simulink model "VehicleDynamics_PathPlanning"  (R2023a)
settings: Solver=FixedStepAuto  StartTime=0.0  StopTime=150  FixedStep=1e-3  RelTol=1e-3
PreLoadFcn:
  | addpath(genpath(pwd));
  | 
  | % ======================================================================= %
  | %% Physics Paramters
  | 
  | g = 9.81;           % [m/s2]
  | rho_air = 1.2;      % [kg/m3]
  | 
  | % ======================================================================= %
  | %% Tire Paramters
  | 
  | mu = 1;           % [-]
  | 
  | B_f = 3.12;
  | B_r = 2.91;
  | C_f = 2.23;
  | C_r = 2.23;
  | D_f = 0.72;
  | D_r = 1.21;
  | E_f = 0.23;
  | E_r = 0.92;
  | 
  | % ======================================================================= %
  | %% Motor Paramters
  | 
  | P_max = 7.6*100;        % [W]
  | 
  | w_l = 1000;           % [RPM]
  | 
  | Motor_Param.eDrivetrain       = 0.8*0.8*0.3;    % [-] %  \eta_i*\eta_d*correction_term
  | 
  | GR1 = 3.3250;         % 84/48*38/20
  | GR2 = 2.90;
  | 
  | % ======================================================================= %
  | %% Car Paramters
  | 
  | widthCar           = 0.31;           % [m]
  | heightCar          = 0.115;          % [m]
  | C_Drag             = 0.7;            % [m]
  | 
  | Car_Param.lTrackWidth         = 0.165;          % [m]
  | l_wb          = 0.3070;           % [m]
  | 
  | mWheel               = 0.03;           % [kg]
  | rWheel               = 0.03;           % [m]
  | I_wheel              = 2.0760e-05;     % [kgm2] % 1/2*mWheel*(rWheel^2+0.022^2)
  | reffWheel            = 0.1885;         % [m]    % rWheel*2*pi
  | 
  | mCar                = 3.31;            % [kg]   % car mass
  | I_z                 = 0.09;            % [kgm2] % 1/12*mCar*(lTrackWidth^2+lWheelbase^2)
  | 
  | h_cg     = 0.02;           % [m]
  | 
  | % ======================================================================= %
  | %% Track Select
  | 
  | NTrack = 1;  % Austin Min Curv
  | % NTrack = 2;  % Austin Shortest Path
  | 
  | % NTrack = 3;  % Silverstone Min Curv
  | % NTrack = 4;  % Silverstone Shortest Path
  | 
  | run TrackData.m
  | Track_Param.rTrajOpt = 0.005; %0.005;
  | 
  | % ======================================================================= %
  | %% Offline Trajectory Optimization
  | 
  | % run Trajectory_Optimizer.m
  | % Track_Param.xTrack=xTraj;
  | % Track_Param.yTrack=yTraj;
StopFcn:
  | Data1=out.CarPosition.Data;
  | 
  | figure(2)
  | cmap = colormap(jet);
  | s=scatter(Data1(:,1),Data1(:,2),0.1,Data1(:,4),'.');
  | c=colorbar;
  | ylabel(c,'v_{Car} (m/s)')
  | 
  | hold on
  | plot(xCentre, yCentre, 'k')
  | plot(xRightside,yRigthside,'k--')
  | k=plot(xLeftside ,yLeftside ,'k--');
  | sf=plot(xStartLine,yStartLine,'k-.');
  | 
  | s.Annotation.LegendInformation.IconDisplayStyle = 'off';
  | k.Annotation.LegendInformation.IconDisplayStyle = 'off';
  | sf.Annotation.LegendInformation.IconDisplayStyle = 'off';
  | legend('Track centerline','Track limits')
  | axis off
  | text(0.5,-5,'S/F\rightarrow','HorizontalAlignment','center')
  | % title('Car position and velocity')
  | 
  | clear Data1 cmap s c k sf
values from neighbouring files (symbols this model uses):
  A_frontal = 0.03565    [PathPlanningFinal.mat]
  C_drag = 0.7    [PathPlanningFinal.mat]
  C_RR = 0.01    [PathPlanningFinal.mat]
  eDriveTrain = 0.192    [PathPlanningFinal.mat]
  l_f = 0.162    [PathPlanningFinal.mat]
  l_r = 0.145    [PathPlanningFinal.mat]
  xStartLine = [-0.53 -0.53]    [PathPlanningFinal.mat]    (also in TrackData.m = [X(1),X(1)])
  xTraj = [-3.58492023158 -0.667650571356 2.24958592115 5.16684606266 8.08415362212 11.0015140612 13.9188994094 16.8363143954 19.7537503159 22.6711684367 25.5885689606 28.505984703 ... (1500 elements, 1500x1)]    [PathPlanningFinal.mat]
  yStartLine = [-3.75 3.75]    [PathPlanningFinal.mat]    (also in TrackData.m = Y(1)+1.5*[-lHalfTrackWidth,lHalfTrackWidth])
  yTraj = [-1.92786957575 -4.15585802925 -6.3838214679 -8.6118036214 -10.8398229653 -13.0678839828 -15.2959656084 -17.5240717548 -19.7521960674 -21.9803092429 -24.2084117195 -26.4365288431 ... (1500 elements, 1500x1)]    [PathPlanningFinal.mat]
libraries: simulink x5, dspfdesign x2, drivingvehiclecontroller x1
settings Model: Creator=Rakshit Jangid  LastModifiedBy=Rakshit Jangid
settings DataIOCC: SaveState=on
settings ModelReferenceCC: UpdateModelReferenceTargets=IfOutOfDate  EnableRefExpFcnMdlSchedulingChecks=on
settings RTWCC: BuildConfiguration=Faster Runs

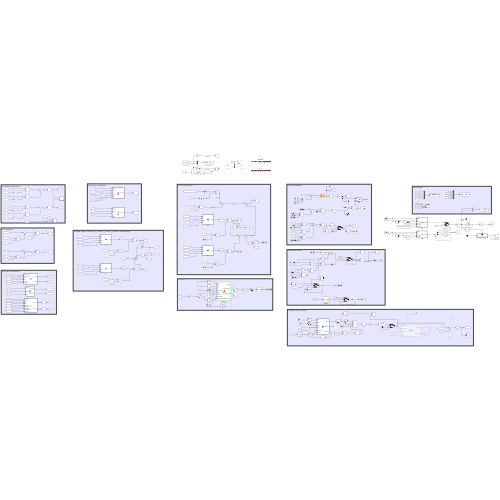
[thumbnail: Simulink's stored preview of the top-level diagram]
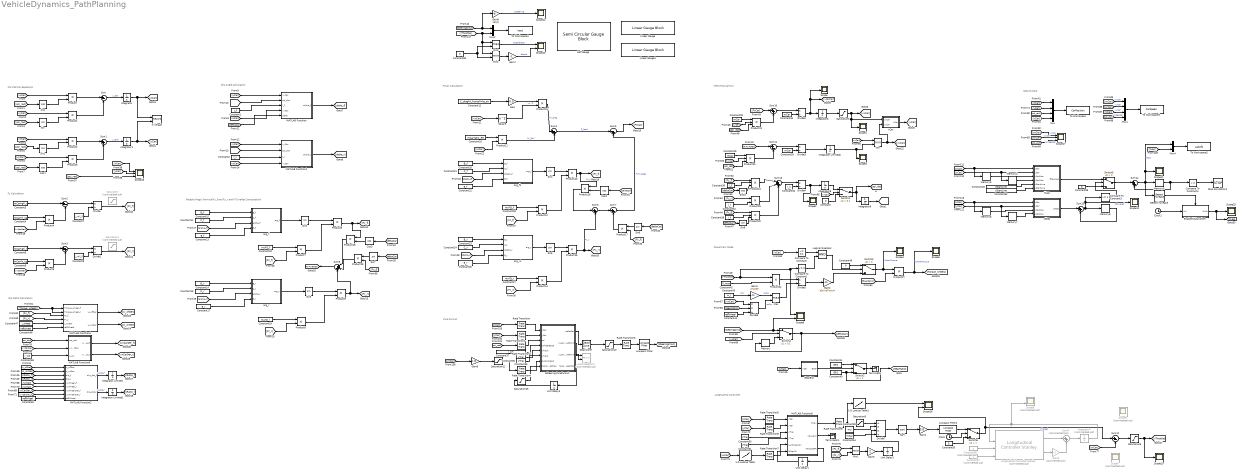
== system VehicleDynamics_PathPlanning ==
  note: Data Output
  note: Pure Pursuit
  note: Longitudinal Controller
  note: Powertrain Model
  note: Vehicle Dynamics
  note: FxCar Calculation
  note: Slip Ratio Calculation
  note: Pacejka Magic Formula(Fy_f and Fy_r and FyTyreNet Computation)
  note: Fz Calculation
  note: Slip Angle Calculation
  note: Car Position Equations
  1-D Lookup Table : Lookup_n-D  NumberOfTableDimensions=1  BreakpointsForDimension1=[7.5, 10, 15, 20]  Table=[5, 10, 25, 40]  ExtrapMethod=Clip  InternalRulePriority=Speed  RndMeth=Simplest
  1-D Lookup Table1 : Lookup_n-D  NumberOfTableDimensions=1  BreakpointsForDimension1=[0,0.04,0.1,0.2,0.3,0.5]*1  Table=[20, 10, 9, 6, 5, 4]  ExtrapMethod=Clip  InternalRulePriority=Speed  RndMeth=Simplest
  Clock : Clock
  Clock1 : Clock
  Compare To Constant : simulink/Logic and Bit Operations/Compare To Constant  relop=<=  const=0.1  OutDataTypeStr=boolean
  Compare To Constant1 : simulink/Logic and Bit Operations/Compare To Constant  relop=<=  const=0  OutDataTypeStr=boolean
  Compare To Constant3 : simulink/Logic and Bit Operations/Compare To Constant  relop=>=  const=1  OutDataTypeStr=boolean
  Compare To Constant4 : simulink/Logic and Bit Operations/Compare To Constant  relop=>  const=2  OutDataTypeStr=boolean
  Constant{,46,59..60} (4 alike) : Constant  Value=0
  Constant1 : Constant  Value=l_f
  Constant10 : Constant  Value=B_f
  Constant11 : Constant  Value=C_f
  Constant12 : Constant  Value=C_drag*A_frontal*rho_air
  Constant13 : Constant  Value=E_f
  Constant14 : Constant  Value=B_r
  Constant15 : Constant  Value=C_r
  Constant16 : Constant  Value=mCar*g*C_RR
  Constant17 : Constant  Value=E_r
  Constant18 : Constant  Value=mu*D_f
  Constant19 : Constant  Value=mu*D_r
  Constant2 : Constant  Value=l_r
  Constant20 : Constant  Value=B_f
  Constant21 : Constant  Value=C_f
  Constant22 : Constant  Value=E_f
  Constant23 : Constant  Value=B_r
  Constant24 : Constant  Value=C_r
  Constant25 : Constant  Value=E_r
  Constant26 : Constant  Value=mu*D_f
  Constant27 : Constant  Value=mu*D_r
  Constant{28..29,33..34,54} (5 alike) : Constant  Value=mCar
  Constant3 : Constant  Value=mCar*g*l_r
  Constant30 : Constant  Value=l_f
  Constant31 : Constant  Value=l_r
  Constant32 : Constant  Value=I_z
  Constant35 : Constant  Value=xTraj
  Constant36 : Constant  Value=yTraj
  Constant37 : Constant  Value=l_wb
  Constant38 : Constant  Value=l_f
  Constant4 : Constant  Value=mCar*h_cg
  Constant40 : Constant  Value=GR1
  Constant41 : Constant  Value=GR2
  Constant42 : Constant  Value=P_max
  Constant43 : Constant  Value=w_l
  Constant44 : Constant  Value=reffWheel
  Constant47 : Constant  Value=I_wheel
  Constant48 : Constant  Value=reffWheel
  Constant49 : Constant  Value=xStartLine
  Constant5 : Constant  Value=reffWheel
  Constant50 : Constant  Value=xTraj
  Constant51 : Constant  Value=yTraj
  Constant52 : Constant  Value=yStartLine
  Constant53 : Constant  Value=mu
  Constant55 : Constant  Value=5
  Constant56 : Constant  Commented=on
  Constant57 : Constant  Commented=on  Value=0
  Constant58 : Constant  Value=l_wb
  Constant6 : Constant  Value=mCar*g*l_f
  Constant7 : Constant  Value=l_r+l_f
  Constant8 : Constant  Value=mCar*h_cg
  Constant9 : Constant  Value=l_r+l_f
  Cos{,1..3} (4 alike) : Trigonometry  Operator=cos
  Dead Zone : DeadZone  LowerValue=-0.5*pi/180  UpperValue=0.5*pi/180
  Detect Increase : simulink/Logic and Bit Operations/Detect Increase  vinit=0.0  OutDataTypeStr=boolean
  Divide{,1..5} (6 alike) : Product  Inputs=*/
  Divide6 : Product  Inputs=**/
  Divide7 : Product  Inputs=/**/
  Enabled Subsystem : Subsystem  TreatAsAtomicUnit=on
  Gain : Gain  Gain=0.5
  Gain1 : Gain  Gain=2*pi/60
  Gain2 : Gain  Gain=eDriveTrain/4
  Gain3 : Gain  Gain=2
  Gain4 : Gain  Gain=0.8
  Gain5 : Gain  Commented=on  Gain=-1
  Gain6 : Gain  Gain=0.25
  Gain7 : Gain  Gain=-1
  Gain8 : Gain  Gain=180/pi
  GearBox : Stateflow chart  TreatAsAtomicUnit=on
  Half Gauge : SemiCircularGaugeBlock  LabelPosition=Bottom  ScaleMin=-5  ScaleMax=5
  Integrator{,1,6,8..9} (5 alike) : Integrator
  Integrator Limited : Integrator  LimitOutput=on  UpperSaturationLimit=10*pi/180  LowerSaturationLimit=-10*pi/180
  Integrator Limited1 : Integrator  LimitOutput=on  UpperSaturationLimit=10*pi/180  LowerSaturationLimit=-10*pi/180
  Integrator Limited2 : Integrator  LimitOutput=on  UpperSaturationLimit=1  LowerSaturationLimit=-1
  Integrator4 : Integrator  Commented=on
  Linear Gauge : LinearGaugeBlock  ScaleMax=1
  Linear Gauge1 : LinearGaugeBlock  ScaleMax=1
  Logical Operator : Logic  AllPortsSameDT=off  OutDataTypeStr=boolean
  Longitudinal Controller Stanley : drivingvehiclecontroller/Longitudinal Controller Stanley  Commented=on  Kp=2.5  Ki=1  SampleTime=0.05  MaxAcceleration=3  MaxDeceleration=6
  LookAheadPoint : Record  Commented=on  FileSettingsInternal="{\"entries\":[{\"content\":{\"excelSettings\":{\"content\":{},\"type\":\"Streamout.ExcelSettings\"}},\"type\":\"Streamout.FileSettingStorage\",\"uuid\":\"\"}],\"packageUris\":[\"http:\\/\\/schema.mathworks.com\\/mf0\\/streamout_blocks\\/R2020a\"],\"version\":\"1.0\"}"  Layout=[1 1]  SignalsInternal="{\"entries\":[{\"content\":{\"signals\":[{\"content\":{\"blockPath\":[],\"dimensions\":[1],\"domain\":\"\",\"lineColor\":\"#a2142f\",\"plots\":[1],\"port\":1,\"signalID\":34,\"signalName\":\"XY Graph:1\"},\"type\":\"RecordBlkView.Signal\",\"uuid\":\"\"},{\"content\":{\"blockPath\":[],\"dimensions\":[1],\"domain\":\"\",\"lineColor\":\"#139fff\",\"plots\":[1],\"port\":2,\"signalID\":37,\"signalName\":\"XY Graph:2\"},\"type\":\"RecordBlkView.Signal\",\"uuid\":\"\"}]},\"type\":\"RecordBlkView.InputSignals\",\"uuid\":\"\"}],\"packageUris\":[\"http:\\/\\/schema.mathworks.com\\/mf0\\/streamout_blocks\\/R2020a\"],\"version\":\"1.0\"}"  VisualizationBindings="{\"xyplotplugin\":{\"info\":[{\"series\":[{\"bindingParametersList\":[{\"parameter\":\"X-Axis\",\"signalID\":34,\"signalName\":\"XY Graph:1\"},{\"parameter\":\"Y-Axis\",\"signalID\":37,\"signalName\":\"XY Graph:2\"}],\"seriesID\":34788}],\"subplotID\":1}]}}"  CompatibilityTag=XY  st=-1
  Lowpass Filter : dspfdesign/Lowpass Filter  FilterType=FIR  DesignForMinimumOrder=on  FilterOrder=50  PassbandFrequency=50  StopbandFrequency=100  PassbandRipple=0.1  StopbandAttenuation=50  SampleRateMode=Specify on dialog  SampleRate=1000  SimulateUsing=Interpreted execution  roundingMode=Floor  coeffsDataTypeStr=fixdt(1,16)
  Lowpass Filter2 : dspfdesign/Lowpass Filter  FilterType=FIR  DesignForMinimumOrder=on  FilterOrder=50  PassbandFrequency=2  StopbandFrequency=10  PassbandRipple=0.1  StopbandAttenuation=50  SampleRateMode=Specify on dialog  SampleRate=1000  SimulateUsing=Interpreted execution  roundingMode=Floor  coeffsDataTypeStr=fixdt(1,16)
  MATLAB Function : MATLAB Function  TreatAsAtomicUnit=on
  MATLAB Function1 : MATLAB Function  TreatAsAtomicUnit=on
  MATLAB Function2 : MATLAB Function  TreatAsAtomicUnit=on
  MATLAB Function4 : MATLAB Function  TreatAsAtomicUnit=on
  MATLAB Function5 : MATLAB Function  TreatAsAtomicUnit=on
  MATLAB Function6 : MATLAB Function  TreatAsAtomicUnit=on
  Max : MinMax  Function=max  Inputs=2
  Memory{,3..4,6..8} (6 alike) : Memory
  Memory5 : Memory  InitialCondition=1
  Min : MinMax  Inputs=2
  Min1 : MinMax  Inputs=2
  Min2 : MinMax  Inputs=2
  Min3 : MinMax  Function=max  Inputs=2
  Mux : Mux
  Mux1 : Mux
  Mux2 : Mux  Inputs=2
  Mux4 : Mux  Inputs=2
  NLap : MATLAB Function  TreatAsAtomicUnit=on
  Product{,1..19,22,25,27} (23 alike) : Product
  Product{20..21,23..24} (4 alike) : Product  Inputs=3
  Rate Transition{,1..2,4..7} (7 alike) : RateTransition  OutPortSampleTime=0.01
  Rate Transition3 : RateTransition  OutPortSampleTime=0.001
  Rate Transition8 : RateTransition  OutPortSampleTime=0.001
  Saturation : Saturate  Commented=on  UpperLimit=mCar*g  LowerLimit=-mCar*g/2
  Saturation1 : Saturate  Commented=on  UpperLimit=mCar*g  LowerLimit=-mCar*g/2
  Saturation10 : Saturate  UpperLimit=26*pi/180  LowerLimit=-26*pi/180
  Saturation12 : Saturate  UpperLimit=5  LowerLimit=1
  Saturation15 : Saturate  UpperLimit=100  LowerLimit=1
  Saturation3 : Saturate  UpperLimit=inf  LowerLimit=0
  Saturation5 : Saturate  UpperLimit=inf  LowerLimit=0.01
  Saturation6 : Saturate  UpperLimit=1  LowerLimit=-1
  Scope{,1..5,10..12,14,25} (11 alike) : Scope
  Scope13 : Scope  NumInputPorts=2
  Scope15 : Scope  NumInputPorts=3
  Scope16 : Scope  NumInputPorts=2
  Scope17 : Scope  NumInputPorts=3
  Scope6 : Scope  NumInputPorts=2
  Scope7 : Scope  Commented=on
  Scope8 : Scope  Commented=on  NumInputPorts=2
  Scope9 : Scope  Commented=on  NumInputPorts=2
  Sin{,1..8} (9 alike) : Trigonometry
  Sin10 : Trigonometry  Operator=cos
  Sqrt : Sqrt  IntermediateResultsDataTypeStr=double
  Square : Math  Operator=square
  Stop Simulation1 : Stop
  Sum{,2,7,11..12} (5 alike) : Sum  Inputs=|+-
  Sum{1,3..4,6,10,14..15} (7 alike) : Sum  Inputs=|++
  Sum13 : Sum  Inputs=|+-+
  Sum5 : Sum  Inputs=|-+
  Sum8 : Sum  Inputs=|+++
  Sum9 : Sum  Commented=on  Inputs=|++
  Switch1 : Switch  Criteria=u2 > Threshold  Threshold=0.1  SaturateOnIntegerOverflow=off  InputSameDT=off
  Switch2 : Switch  Criteria=u2 > Threshold  Threshold=1  SaturateOnIntegerOverflow=off  InputSameDT=off
  Switch3 : Switch  Criteria=u2 > Threshold  SaturateOnIntegerOverflow=off  InputSameDT=off
  Switch4 : Switch  Criteria=u2 > Threshold  Threshold=0.1  SaturateOnIntegerOverflow=off  InputSameDT=off
  Switch5 : Switch  Criteria=u2 > Threshold  SaturateOnIntegerOverflow=off  InputSameDT=off
  Switch6 : Switch  Criteria=u2 > Threshold  Threshold=1  SaturateOnIntegerOverflow=off  InputSameDT=off
  Terminator : Terminator
  Terminator1 : Terminator
  To Workspace : ToWorkspace  VariableName=CarPosition  SaveFormat=Timeseries  SampleTime=-1
  To Workspace1 : ToWorkspace  VariableName=Input  SaveFormat=Timeseries  SampleTime=-1
  To Workspace2 : ToWorkspace  VariableName=LapInfo  SaveFormat=Timeseries  SampleTime=-1
  To Workspace3 : ToWorkspace  VariableName=CarSpeed  SaveFormat=Timeseries  SampleTime=-1
  Unit Delay1 : UnitDelay  SampleTime=-1  HasFrameUpgradeWarning=on
  Unit Delay2 : UnitDelay  SampleTime=0.001  HasFrameUpgradeWarning=on
  Unit Delay3 : UnitDelay  InitialCondition=1  SampleTime=-1  HasFrameUpgradeWarning=on
  XY Graph : Record  FileSettingsInternal="{\"entries\":[{\"content\":{\"excelSettings\":{\"content\":{},\"type\":\"Streamout.ExcelSettings\"}},\"type\":\"Streamout.FileSettingStorage\",\"uuid\":\"\"}],\"packageUris\":[\"http:\\/\\/schema.mathworks.com\\/mf0\\/streamout_blocks\\/R2020a\"],\"version\":\"1.0\"}"  Layout=[1 1]  SignalsInternal="{\"entries\":[{\"content\":{\"signals\":[{\"content\":{\"blockPath\":[],\"dimensions\":[1,1],\"domain\":\"\",\"lineColor\":\"#a2142f\",\"plots\":[1],\"port\":1,\"sid\":[\"\"],\"signalID\":628,\"signalName\":\"Integrator\"},\"type\":\"RecordBlkView.Signal\",\"uuid\":\"\"},{\"content\":{\"blockPath\":[],\"dimensions\":[1,1],\"domain\":\"\",\"lineColor\":\"#139fff\",\"plots\":[1],\"port\":2,\"sid\":[\"\"],\"signalID\":632,\"signalName\":\"Integrator1\"},\"type\":\"RecordBlkView.Signal\",\"uuid\":\"\"}]},\"type\":\"RecordBlkView.InputSignals\",\"uuid\":\"\"}],\"packageUris\":[\"http:\\/\\/schema.mathworks.com\\/mf0\\/streamout_blocks\\/R2020a\"],\"version\":\"1.0\"}"  VisualizationBindings="{\"xyplotplugin\":{\"info\":[{\"series\":[{\"bindingParametersList\":[{\"parameter\":\"X-Axis\",\"signalID\":628,\"signalName\":\"Integrator\"},{\"parameter\":\"Y-Axis\",\"signalID\":632,\"signalName\":\"Integrator1\"}],\"seriesID\":23987}],\"subplotID\":1}]}}"  CompatibilityTag=XY
  aSteering PurePursuit : MATLAB Function  TreatAsAtomicUnit=on
  arg_f : MATLAB Function  TreatAsAtomicUnit=on
  arg_f1 : MATLAB Function  TreatAsAtomicUnit=on
  arg_r : MATLAB Function  TreatAsAtomicUnit=on
  arg_r1 : MATLAB Function  TreatAsAtomicUnit=on
  sStep : MATLAB Function  TreatAsAtomicUnit=on
  vCar : MATLAB Function  TreatAsAtomicUnit=on
  wires:
  [vxCar] -> Product/1
  [psi_rad] -> Cos/1
  Cos/1 -> Product/2
  Product/1 -> Sum/1
  [vyCar] -> Product1/1
  Sin/1 -> Product1/2
  Product1/1 -> Sum/2
  [psi_rad] -> Sin/1
  Sum/1 -> Integrator/1  "x_dot"
  Integrator/1 -> XY Graph/1, [xCar]
  [vxCar] -> Product2/1
  [psi_rad] -> Sin1/1
  Sin1/1 -> Product2/2
  [vyCar] -> Product3/1
  [psi_rad] -> Cos1/1
  Cos1/1 -> Product3/2
  Product2/1 -> Sum1/1
  Product3/1 -> Sum1/2
  Sum1/1 -> Integrator1/1  "y_Dot"
  Integrator1/1 -> XY Graph/2, [yCar]
  Constant1/1 -> MATLAB Function/3(l_f)
  [vxCar] -> MATLAB Function/4(vxCar)
  [vyCar] -> MATLAB Function/1(vyCar)
  [psi_dot] -> MATLAB Function/2(psi_dot)
  [deltaCar] -> MATLAB Function/5(delta)
  MATLAB Function/1(alpha_f) -> [alpha_f]
  [vyCar] -> MATLAB Function1/1(vyCar)
  [psi_dot] -> MATLAB Function1/2(psi_dot)
  Constant2/1 -> MATLAB Function1/3(l_r)
  [vxCar] -> MATLAB Function1/4(vxCar)
  MATLAB Function1/1(alpha_r) -> [alpha_r]
  Constant3/1 -> Sum2/1
  Constant4/1 -> Product4/1
  [vxCarDer] -> Product4/2
  Product4/1 -> Sum2/2
  Sum2/1 -> Divide/1
  Constant7/1 -> Divide/2
  Divide/1 -> [Fz_f]
  Constant6/1 -> Sum3/1
  Constant8/1 -> Product5/1
  [vxCarDer] -> Product5/2
  Product5/1 -> Sum3/2
  Sum3/1 -> Divide1/1
  Constant9/1 -> Divide1/2
  Divide1/1 -> [Fz_r]
  Constant10/1 -> arg_f/1(B_f)
  Constant11/1 -> arg_f/2(C_f)
  [alpha_f] -> arg_f/3(alpha_f)
  arg_f/1(arg_f) -> Sin2/1
  Sin2/1 -> Product6/1
  Constant18/1 -> Product7/1
  [Fz_f] -> Product7/2
  Product7/1 -> Product6/2
  Product6/1 -> Product18/1, [Fy_f]
  Constant14/1 -> arg_r/1(B_r)
  Constant15/1 -> arg_r/2(C_r)
  [alpha_r] -> arg_r/3(alpha_r)
  arg_r/1(arg_r) -> Sin3/1
  Constant19/1 -> Product8/1
  [Fz_r] -> Product8/2
  Product8/1 -> Product9/2
  Sin3/1 -> Product9/1
  Product9/1 -> Sum8/3, [Fy_r]
  Constant13/1 -> arg_f/4(E_f)
  Constant17/1 -> arg_r/4(E_r)
  [vxCar] -> Square/1
  Square/1 -> Product10/2  "vx^2"
  Constant12/1 -> Gain/1
  Gain/1 -> Product10/1
  Product10/1 -> Sum4/1  "Fx_drag"
  Constant16/1 -> Product11/1
  [vxCar] -> Product11/2
  Product11/1 -> Sum4/2  "Fx_Roll"
  Sum4/1 -> Sum5/1  "F_load"
  [w_wfDer] -> MATLAB Function2/1(w_wfDer)
  MATLAB Function2/1(slip_dot_f) -> Integrator Limited/1  "s_dot_f"
  Integrator Limited/1 -> [sRatio_f]
  [w_wrDer] -> MATLAB Function2/2(w_wrDer)
  MATLAB Function2/2(slip_dot_r) -> Integrator Limited1/1  "s_dot_r"
  Integrator Limited1/1 -> [sRatio_r]
  Constant22/1 -> arg_f1/4(E_f)
  Constant21/1 -> arg_f1/2(C_f)
  Constant20/1 -> arg_f1/1(B_f)
  [sRatio_f] -> arg_f1/3(sRatio_f)
  arg_f1/1(arg_f) -> Sin4/1
  Constant26/1 -> Product12/1
  Product12/1 -> Product13/2
  [Fz_f] -> Product12/2
  Sin4/1 -> Product13/1
  Product13/1 -> [Fx_f], Product16/1  "Fx_f"
  Sin5/1 -> Product15/1
  Product15/1 -> Sum6/2, [Fx_r]  "Fx_r"
  [Fz_r] -> Product14/2
  Constant27/1 -> Product14/1
  Product14/1 -> Product15/2
  arg_r1/1(arg_r) -> Sin5/1
  Constant23/1 -> arg_r1/1(B_r)
  Constant25/1 -> arg_r1/4(E_r)
  [sRatio_r] -> arg_r1/3(sRatio_r)
  Constant24/1 -> arg_r1/2(C_r)
  Sum6/1 -> Sum7/1
  Sum5/1 -> [FxCar]
  Cos2/1 -> Product16/2
  [deltaCar] -> Cos2/1
  Product16/1 -> Sum6/1
  [deltaCar] -> Sin6/1
  Sin6/1 -> Product17/1
  [Fy_f] -> Product17/2
  Product17/1 -> Sum7/2
  Sum7/1 -> Sum5/2  "FxTyreNet"
  [deltaCar] -> Cos3/1
  Cos3/1 -> Product18/2
  Sin7/1 -> Product19/1
  [deltaCar] -> Sin7/1
  Product19/1 -> Sum8/2
  [Fx_f] -> Product19/2
  Product18/1 -> Sum8/1
  Sum8/1 -> [FyTyreNet]
  Constant28/1 -> Product21/1
  [vyCar] -> Product21/2
  [psi_dot] -> Product21/3
  Product21/1 -> Sum10/2
  Sum10/1 -> Divide2/1
  Constant34/1 -> Divide2/2
  Divide2/1 -> Scope/1, [vxCarDer], Integrator6/1
  Integrator6/1 -> Saturation3/1
  Saturation3/1 -> vCar/1(vxCar), Scope1/1, [vxCar]
  Constant29/1 -> Product23/1
  Integrator Limited2/1 -> Min/2, Scope3/1
  [vxCar] -> Product23/2
  Sum11/1 -> Divide3/1
  Divide3/1 -> Integrator Limited2/1
  Constant33/1 -> Divide3/2
  [psi_dot] -> Product23/3
  Product23/1 -> Sum11/2
  [Fy_f] -> Product24/1
  Constant30/1 -> Product24/2
  [deltaCar] -> Sin10/1
  Sin10/1 -> Product24/3
  Product24/1 -> Sum13/1
  [Fy_r] -> Product25/1
  Constant31/1 -> Product25/2
  Product25/1 -> Sum13/2
  Sum13/1 -> Divide4/1
  Constant32/1 -> Divide4/2
  Divide4/1 -> Scope2/1, Integrator8/1
  [vxCar] -> Min/1
  Min/1 -> vCar/2(vyCar), [vyCar]
  Integrator9/1 -> [psi_rad]
  [vxCar] -> Switch1/2
  Constant/1 -> Switch1/3
  Integrator8/1 -> Switch1/1
  Switch1/1 -> [psi_dot], Integrator9/1
  [FyTyreNet] -> Sum11/1
  [deltaCar] -> Sin8/1
  [Fx_f] -> Product20/1
  Constant38/1 -> Product20/2
  Sin8/1 -> Product20/3
  Product20/1 -> Sum13/3
  vCar/1(vCar) -> [vCar]
  [vCar] -> GearBox/1(vCar)
  GearBox/1(Gear) -> Switch2/2
  Constant41/1 -> Switch2/1
  Constant40/1 -> [GearRatio], Switch2/3
  [rThrottle] -> Scope6/1, Compare To Constant1/1, Product22/1
  Product22/1 -> Divide5/1
  Max/1 -> Divide5/2
  Constant43/1 -> Gain1/1  "rpm"
  [vxCar] -> Divide6/1
  [GearRatio] -> Divide6/2
  Constant44/1 -> Divide6/3
  Divide6/1 -> Max/2  "rad/s"
  Gain1/1 -> Max/1  "rad/s"
  [vCar] -> Compare To Constant/1
  Compare To Constant/1 -> Logical Operator/1
  Compare To Constant1/1 -> Logical Operator/2
  Logical Operator/1 -> Switch3/2
  Constant46/1 -> Switch3/1
  [Torque_wheels] -> MATLAB Function4/2(Torque_wheel_r), MATLAB Function4/1(Torque_wheel_f)
  [Fx_f] -> MATLAB Function4/3(Fx_f)
  [Fx_r] -> MATLAB Function4/4(Fx_r)
  Constant47/1 -> MATLAB Function4/5(I_wheel)
  Constant48/1 -> MATLAB Function4/6(reffWheel)
  MATLAB Function4/2(w_wrDer) -> [w_wrDer]
  MATLAB Function4/1(w_wfDer) -> [w_wfDer]
  Switch3/1 -> Scope4/1, Product27/1  "MotorTorque"
  [GearRatio] -> Product27/2
  Product27/1 -> Scope5/1, [Torque_wheels]  "WheelTorque"
  Constant5/1 -> MATLAB Function2/9(reffWheel)
  [sRatio_f] -> MATLAB Function2/3(slip_f)
  [sRatio_r] -> MATLAB Function2/4(slip_r)
  [vxCar] -> MATLAB Function2/5(vxWheel_f)
  [vxCar] -> MATLAB Function2/6(vxWheel_r)
  [vxCarDer_f] -> MATLAB Function2/7(vxWheelDer_f)
  [vxCarDer_r] -> MATLAB Function2/8(vxWheelDer_r)
  [SteeringCmd] -> Scope6/2, Switch4/1
  [vxCar] -> Switch4/2
  Switch4/1 -> Memory/1, [deltaCar]
  Memory/1 -> Switch4/3
  [xCar] -> Rate Transition5/1
  [yCar] -> Rate Transition6/1
  Rate Transition5/1 -> MATLAB Function5/1(xCar)
  Rate Transition6/1 -> MATLAB Function5/2(yCar)
  Constant50/1 -> MATLAB Function5/3(xTraj)
  Constant51/1 -> MATLAB Function5/4(yTraj)
  [vxCar] -> 1-D Lookup Table/1
  1-D Lookup Table/1 -> Rate Transition7/1
  Rate Transition7/1 -> MATLAB Function5/5(sAnticipation)
  MATLAB Function5/1(KMax) -> Rate Transition8/1
  MATLAB Function5/3(NClosestPt) -> Unit Delay1/1
  Unit Delay1/1 -> MATLAB Function5/6(NPrevPt)
  MATLAB Function5/2(KCurrent) -> Terminator1/1
  Rate Transition8/1 -> 1-D Lookup Table1/1, Saturation5/1
  Saturation5/1 -> Divide7/1
  [Fz_f] -> Min1/1
  [Fz_r] -> Min1/2
  Min1/1 -> Gain3/1
  Gain3/1 -> Unit Delay2/1
  Unit Delay2/1 -> Divide7/3
  Constant53/1 -> Divide7/2
  Constant54/1 -> Divide7/4
  Divide7/1 -> Sqrt/1
  Sqrt/1 -> Gain4/1
  Gain4/1 -> Lowpass Filter2/1
  Lowpass Filter2/1 -> Switch6/1
  Clock/1 -> Switch6/2
  Constant55/1 -> Switch6/3
  Switch6/1 -> Scope16/2, Sum12/1  "vTarget"
  Constant56/1 -> Longitudinal Controller Stanley/3
  Constant57/1 -> Longitudinal Controller Stanley/4
  Longitudinal Controller Stanley/1 -> Sum9/1
  Longitudinal Controller Stanley/2 -> Gain5/1
  Sum9/1 -> Integrator4/1
  Gain5/1 -> Sum9/2
  Integrator4/1 -> Scope8/2, Longitudinal Controller Stanley/2
  Sum12/1 -> Saturation6/1
  Saturation6/1 -> Scope10/1, [rThrottle]
  [psi_dot] -> MATLAB Function6/1(psi_dot)
  [vxCarDer] -> MATLAB Function6/2(vxCarDer)
  Constant58/1 -> MATLAB Function6/3(l_wb)
  MATLAB Function6/2(vxCarDer_r) -> [vxCarDer_r]
  MATLAB Function6/1(vxCarDer_f) -> [vxCarDer_f]
  Switch2/1 -> Terminator/1
  aSteering PurePursuit/2(xLookAheadPoint) -> LookAheadPoint/1
  Constant37/1 -> aSteering PurePursuit/4(lWheelBase)
  [psi_rad] -> Rate Transition2/1
  Rate Transition2/1 -> aSteering PurePursuit/3(psi)
  Rate Transition1/1 -> aSteering PurePursuit/2(yCar)
  Constant36/1 -> aSteering PurePursuit/6(yTrack)
  Dead Zone/1 -> Saturation10/1
  Constant35/1 -> aSteering PurePursuit/5(xTrack)
  Lowpass Filter/1 -> [SteeringCmd]
  aSteering PurePursuit/4(NLookAheadOpt) -> Unit Delay3/1
  Rate Transition/1 -> aSteering PurePursuit/1(xCar)
  aSteering PurePursuit/1(deltaCar) -> Dead Zone/1
  Saturation15/1 -> aSteering PurePursuit/8(NLookAheadPrev)
  Saturation10/1 -> Rate Transition3/1
  Gain6/1 -> Saturation12/1
  [vxCar] -> Gain6/1
  [xCar] -> Rate Transition/1
  [yCar] -> Rate Transition1/1
  Rate Transition3/1 -> Lowpass Filter/1
  Rate Transition4/1 -> aSteering PurePursuit/7(sLookAhead)
  aSteering PurePursuit/3(yLookAheadPoint) -> LookAheadPoint/2
  Saturation12/1 -> Rate Transition4/1
  Unit Delay3/1 -> Saturation15/1
  [FxCar] -> Sum10/1
  [yCar] -> Memory7/1, sStep/2(yCar)
  Memory4/1 -> NLap/4(yCarPrev)
  Memory5/1 -> Compare To Constant4/1, Sum14/2
  Constant52/1 -> NLap/6(yStartLine)
  Constant49/1 -> NLap/5(xStartLine)
  [xCar] -> Memory6/1, sStep/1(xCar)
  Memory7/1 -> sStep/4(yCarPrev)
  [xCar] -> Memory3/1, NLap/1(xCar)
  Constant59/1 -> Switch5/3
  [yCar] -> Memory4/1, NLap/2(yCar)
  Memory6/1 -> sStep/3(xCarPrev)
  Clock1/1 -> Enabled Subsystem/1(In1)
  NLap/1(BNewLap) -> Switch5/1
  Memory8/1 -> Sum15/2
  Detect Increase/1 -> Enabled Subsystem/Enable
  Sum15/1 -> Memory8/1, Scope12/1, Compare To Constant3/1  "sCovered"
  Memory3/1 -> NLap/3(xCarPrev)
  Compare To Constant4/1 -> Stop Simulation1/1
  sStep/1(sStep) -> Sum15/1
  Enabled Subsystem/1(Out1) -> [tLap], Scope25/1
  Switch5/1 -> Sum14/1
  Compare To Constant3/1 -> Switch5/2
  Sum14/1 -> Mux4/1, Scope11/1, Detect Increase/1, Memory5/1  "NLap"
  [tLap] -> Mux4/2
  Mux4/1 -> To Workspace2/1
  [vxCar] -> Sum12/2
  Mux2/1 -> To Workspace1/1
  Min3/1 -> Scope13/1  "rAccelerator"
  Gain8/1 -> Scope14/1  "aSteering"
  Gain7/1 -> Scope13/2  "rBrake"
  Min2/1 -> Gain7/1
  Constant60/1 -> Min3/2, Min2/2
  [rThrottle] -> Min2/1, Min3/1, Mux2/2
  [psi_rad] -> Scope15/3
  [xCar] -> Scope15/1
  [yCar] -> Scope15/2
  1-D Lookup Table1/1 -> Scope16/1
  [SteeringCmd] -> Gain8/1, Mux2/1
  [xCar] -> Mux/1
  [yCar] -> Mux/2
  [psi_rad] -> Mux/3
  [vCar] -> Mux/4
  Mux/1 -> To Workspace/1
  [vyCar] -> Scope17/2  "vyCar"
  [vxCar] -> Scope17/1  "vxCar"
  [psi_dot] -> Scope17/3  "omegaCar"
  [vxCar] -> Mux1/1  "vxCar"
  [vyCar] -> Mux1/2  "vyCar"
  [vCar] -> Mux1/3  "vyCar"
  [psi_dot] -> Mux1/4  "omegaCar"
  Mux1/1 -> To Workspace3/1
  Constant42/1 -> Product22/2
  Divide5/1 -> Gain2/1
  Gain2/1 -> Switch3/3

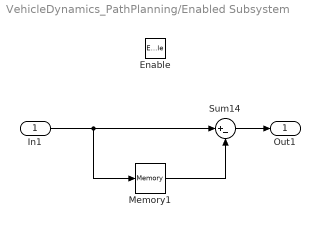
== system VehicleDynamics_PathPlanning/Enabled Subsystem ==
  In1 : Inport
  Enable : EnablePort
  Memory1 : Memory
  Sum14 : Sum  Inputs=|+-
  Out1 : Outport
  wires:
  In1/1 -> Sum14/1, Memory1/1
  Sum14/1 -> Out1/1
  Memory1/1 -> Sum14/2

== matlab function VehicleDynamics_PathPlanning/aSteering PurePursuit ==
  data: xCar input; deltaCar output; yCar input; psi input; lWheelBase input; xTrack input; yTrack input; sLookAhead input; xLookAheadPoint output; yLookAheadPoint output; NLookAheadOpt output; NLookAheadPrev input
function [deltaCar,xLookAheadPoint,yLookAheadPoint,NLookAheadOpt] = aSteering(xCar,yCar,psi,lWheelBase,xTrack,yTrack,sLookAhead,NLookAheadPrev)


NLookAheadOpt=NLookAheadPrev;
sLookAheadOpt=sqrt((xTrack(NLookAheadOpt)-xCar)^2+(yTrack(NLookAheadOpt)-yCar)^2)-sLookAhead;

for N=NLookAheadOpt+1:min(NLookAheadOpt+100,length(xTrack))
    
    NN=N; %mod(N-1,length(xTrack)-1)+1
    
    sTemp=sqrt((xTrack(NN)-xCar)^2+(yTrack(NN)-yCar)^2)-sLookAhead;
    
    if abs(sTemp)<abs(sLookAheadOpt)
        NLookAheadOpt=NN;
        sLookAheadOpt=sTemp;
    end
end

aTemp=atan2((yTrack(NLookAheadOpt)-yCar),(xTrack(NLookAheadOpt)-xCar));
aTemp=mod(aTemp+pi,2*pi)-pi;
aHeadingError=psi-aTemp;

deltaCar=-atan(2*lWheelBase*sin(aHeadingError)/sLookAhead);

xLookAheadPoint=xTrack(NLookAheadOpt);
yLookAheadPoint=yTrack(NLookAheadOpt);

%% Plot

% figure(7)
% hold on
% plot(xTrack(NLookAheadOpt),yTrack(NLookAheadOpt),'k+')
% plot(xCar,yCar,'r+')

== stateflow chart VehicleDynamics_PathPlanning/GearBox ==
  state Gear1
    en:
    Gear = 1;
  state Gear2
    en:
    Gear = 2;
  (default) -> Gear1
  Gear1 -> Gear2 : [vCar>9.5]
  Gear2 -> Gear1 : [vCar<9]
  data: vCar input; Gear output

== matlab function VehicleDynamics_PathPlanning/vCar ==
  data: vxCar input; vCar output; vyCar input
function vCar = fcn(vxCar, vyCar)

vCar = sqrt((vxCar)^2 + (vyCar)^2);

end

== matlab function VehicleDynamics_PathPlanning/MATLAB Function4 ==
  data: Torque_wheel_f input; Torque_wheel_r input; Fx_f input; Fx_r input; I_wheel input; reffWheel input; w_wfDer output; w_wrDer output
function [w_wfDer, w_wrDer] = fcn(Torque_wheel_f, Torque_wheel_r, Fx_f, Fx_r, I_wheel, reffWheel)

w_wfDer = (1/I_wheel)*(Torque_wheel_f-reffWheel*Fx_f);

w_wrDer = (1/I_wheel)*(Torque_wheel_r-reffWheel*Fx_r);

end

== matlab function VehicleDynamics_PathPlanning/MATLAB Function5 ==
  data: KMax output; KCurrent output; xCar input; NClosestPt output; yCar input; xTraj input; yTraj input; sAnticipation input; NPrevPt input
function [KMax, KCurrent, NClosestPt] = fcn(xCar, yCar, xTraj, yTraj, sAnticipation, NPrevPt)

NClosestPt = NPrevPt;

%%

NTemp = max(NClosestPt, 2);
sTemp = sqrt((xTraj(NTemp)-xCar)^2+(yTraj(NTemp)-yCar)^2);

KList = zeros(1, length(xTraj));

while sTemp<sAnticipation && NTemp<length(xTraj)-1

    %Curvature calculation

    A=[xTraj(NTemp-1);yTraj(NTemp-1);0];
    B=[xTraj(NTemp)  ;yTraj(NTemp)  ;0];
    C=[xTraj(NTemp+1);yTraj(NTemp+1);0];
    
    D = cross(B-A,C-A);
    b = norm(A-C);
    c = norm(A-B);
    a = norm(B-C);
    R = a*b*c/2/norm(D);
    
    K=1/R;
    KList(NTemp)=K;
    
    % Next point
    
    NTemp = NTemp+1;
    sTemp = sTemp+sqrt((xTraj(NTemp)-xTraj(NTemp-1))^2+(yTraj(NTemp)-yTraj(NTemp-1))^2);
end

KTemp = maxk(KList, min(3, length(KList)));
KMax = KTemp(min(3, length(KList)));
KCurrent = KList(1);

end

== matlab function VehicleDynamics_PathPlanning/MATLAB Function6 ==
  data: vxCarDer_f output; psi_dot input; vxCarDer input; l_wb input; vxCarDer_r output
function [vxCarDer_f, vxCarDer_r] = fcn(psi_dot, vxCarDer, l_wb)

vxCarDer_f = vxCarDer + psi_dot^2*l_wb/2;
vxCarDer_r = vxCarDer - psi_dot^2*l_wb/2;

end

== matlab function VehicleDynamics_PathPlanning/NLap ==
  data: xCar input; BNewLap output; yCar input; xCarPrev input; yCarPrev input; xStartLine input; yStartLine input
function BNewLap ...
         = NLap(xCar,yCar,...
                xCarPrev,yCarPrev,...
                xStartLine,yStartLine)
BNewLap=0;
            
if xCar==xCarPrev && yCar==yCarPrev
    BNewLap=0;
end

% https://ericleong.me/research/circle-line/

x1=xCar;            y1=yCar;
x2=xCarPrev;        y2=yCarPrev;
x3=xStartLine(1);   y3=yStartLine(1);
x4=xStartLine(2);   y4=yStartLine(2);


a1=y2-y1;           a2=y4-y3;
b1=x1-x2;           b2=x3-x4;
c1=a1*x1+b1*y1;     c2=a2*x3+b2*y3;

d=det([a1,b1;a2,b2]);

if d==0
    BNewLap=0;
end

x=det([c1,b1;c2,b2])/d;
y=det([a1,c1;a2,c2])/d;

if x >= min(x1, x2) && x <= max(x1, x2) ...
   && x >= min(x3, x4) && x <= max(x3, x4) ...
   && y >= min(y1, y2) && y <= max(y1, y2) ...
   && y >= min(y3, y4) && y <= max(y3, y4)

    BNewLap=1;
end

end

== matlab function VehicleDynamics_PathPlanning/sStep ==
  data: xCar input; sStep output; yCar input; xCarPrev input; yCarPrev input
function sStep ...
         = sStep(xCar,yCar,...
                xCarPrev,yCarPrev)

sStep=sqrt((xCar-xCarPrev)^2+(yCar-yCarPrev)^2)

end

== matlab function VehicleDynamics_PathPlanning/MATLAB Function1 ==
  data: vyCar input; alpha_r output; psi_dot input; l_r input; vxCar input
function alpha_r = fcn(vyCar, psi_dot, l_r, vxCar)

alpha_r = -atan((vyCar-(psi_dot*l_r))/vxCar);

end

== matlab function VehicleDynamics_PathPlanning/MATLAB Function ==
  data: vyCar input; alpha_f output; psi_dot input; l_f input; vxCar input; delta input
function alpha_f = fcn(vyCar, psi_dot, l_f, vxCar, delta)

alpha_f = -atan((vyCar+psi_dot*l_f)/vxCar)+delta;

end

== matlab function VehicleDynamics_PathPlanning/arg_f ==
  data: B_f input; arg_f output; C_f input; alpha_f input; E_f input
function arg_f = fcn(B_f, C_f, alpha_f, E_f)

arg_f = C_f*atan(B_f*alpha_f-E_f*(B_f*alpha_f-atan(B_f*alpha_f)));

end

== matlab function VehicleDynamics_PathPlanning/arg_r ==
  data: B_r input; arg_r output; C_r input; alpha_r input; E_r input
function arg_r = fcn(B_r, C_r, alpha_r, E_r)

arg_r = C_r*atan(B_r*alpha_r-E_r*(B_r*alpha_r-atan(B_r*alpha_r)));

end

== matlab function VehicleDynamics_PathPlanning/MATLAB Function2 ==
  data: w_wfDer input; w_wrDer input; slip_f input; slip_r input; slip_dot_f output; vxWheel_f input; vxWheel_r input; vxWheelDer_f input; slip_dot_r output; vxWheelDer_r input; reffWheel input
function [slip_dot_f, slip_dot_r]= fcn(w_wfDer, w_wrDer,...
                                       slip_f, slip_r,...
                                       vxWheel_f, vxWheel_r,...
                                       vxWheelDer_f, vxWheelDer_r,...
                                       reffWheel)

% s_dot_f = (w_wfDer*reff/vxCar)-(w_wf*reff*vxCarDer)/(vxCar*vxCar);
% s_dot_r = (w_wrDer*reff/vxCar)-(w_wr*reff*vxCarDer)/(vxCar*vxCar);

if abs(vxWheel_f)<=1
    slip_dot_f = w_wfDer*reffWheel-vxWheelDer_f*(slip_f+1);
else
    slip_dot_f = w_wfDer*reffWheel/vxWheel_f-vxWheelDer_f/vxWheel_f^2*(slip_f+1);
end

if abs(vxWheel_r)<=1
    slip_dot_r = w_wrDer*reffWheel-vxWheelDer_r*(slip_r+1);
else
    slip_dot_r = w_wrDer*reffWheel/vxWheel_r-vxWheelDer_r/vxWheel_r^2*(slip_r+1);
end

% note that since we are using single track model, hence vxWheel_f and
% vxWheel_r are both equal to vxCar.
                           
end

== matlab function VehicleDynamics_PathPlanning/arg_f1 ==
  data: B_f input; arg_f output; C_f input; sRatio_f input; E_f input
function arg_f = fcn(B_f, C_f, sRatio_f, E_f)

arg_f = C_f*atan((B_f*sRatio_f)-E_f*((B_f*sRatio_f)-atan(B_f*sRatio_f)));

end

== matlab function VehicleDynamics_PathPlanning/arg_r1 ==
  data: B_r input; arg_r output; C_r input; sRatio_r input; E_r input
function arg_r = fcn(B_r, C_r, sRatio_r, E_r)

arg_r = C_r*atan((B_r*sRatio_r)-E_r*((B_r*sRatio_r)-atan(B_r*sRatio_r)));

end
